simulink model "ex4s"  (R2013a)
settings: Solver=ode45  StartTime=0.0  StopTime=10.0  RelTol=1e-3
settings Model: Creator=Edward  LastModifiedBy=Edward

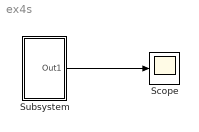
== system ex4s ==
  Scope : Scope
  Subsystem : Subsystem  mask{a=4, b=36}
      mask prompts: a "val a"; b "val b"
      mask Callback a:
      | if str2num(get_param(gcb,'a'))<0
      |     error('negativa!!!')
      | end
      mask Callback b:
      | if str2num(get_param(gcb,'b'))<0
      |     error('negativa!!!')
      | end
  wires:
  Subsystem/1(Out1) -> Scope/1

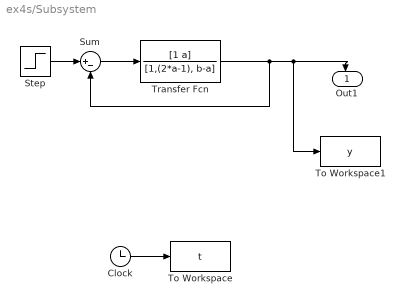
== system ex4s/Subsystem ==
  Clock : Clock
  Step : Step  SampleTime=0
  Sum : Sum  Inputs=|+-
  To Workspace : ToWorkspace  VariableName=t  SampleTime=-1
  To Workspace1 : ToWorkspace  VariableName=y  SampleTime=-1
  Transfer Fcn : TransferFcn  Numerator=[1 a]  Denominator=[1,(2*a-1), b-a]
  Out1 : Outport
  wires:
  Sum/1 -> Transfer Fcn/1
  Step/1 -> Sum/1
  Transfer Fcn/1 -> To Workspace1/1, Out1/1, Sum/2
  Clock/1 -> To Workspace/1
